simulink model "gm_sampleModel1489_sub"  (R2023a)
settings: Solver=VariableStepAuto  StartTime=0.0  StopTime=10.0  RelTol=1e-3
libraries: hdlsllib x3, simulink x1
settings Model: Creator=user1  LastModifiedBy=user1
settings OptimizationCC: BlockReduction=off  ConditionallyExecuteInputs=off
settings DebuggingCC: InheritedTsInSrcMsg=none

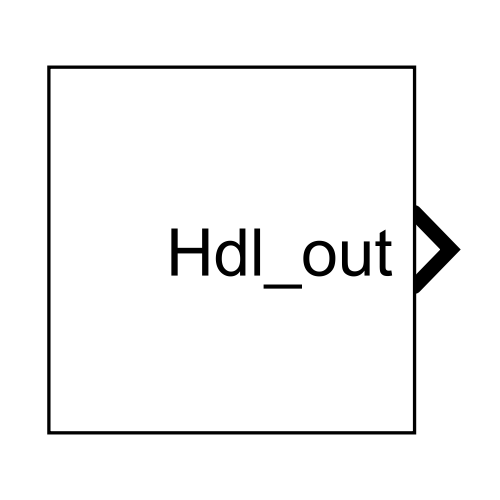
[thumbnail: Simulink's stored preview of the top-level diagram]
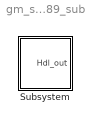
== system gm_sampleModel1489_sub ==
  Subsystem : Subsystem

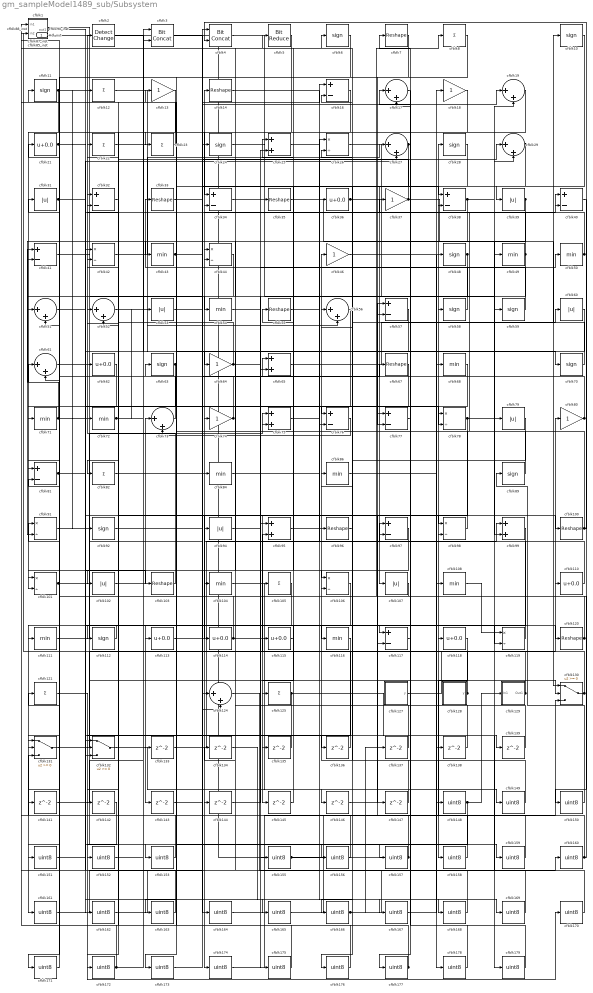
== system gm_sampleModel1489_sub/Subsystem ==
  cfblk1 : Constant  Value=0  OutDataTypeStr=uint8  SampleTime=1
  cfblk{6,10..11,24,28,48,58..59,63,70,89,92,112} (13 alike) : Signum
  cfblk{7,14,33,35,55,67,96,100,103,120} (10 alike) : Reshape
  cfblk{26,42,44,78,91,98,101,106,119} (9 alike) : Product  Inputs=*/  OutDataTypeStr=uint8  RndMeth=Zero  SaturateOnIntegerOverflow=on
  cfblk{31,39,53,60,79,94,102,107} (8 alike) : Abs  OutDataTypeStr=uint8  SaturateOnIntegerOverflow=off
  cfblk{43,49..50,54,68,71..72,84,86,104,108,111,116} (13 alike) : MinMax  OutDataTypeStr=uint8
  cfblk{8,12,22..23,82,105,121,125} (8 alike) : Sum  Inputs=+  OutDataTypeStr=uint8
  cfblk{21,36,62,110,113..115,118} (8 alike) : Bias  Bias=0.0  SaturateOnIntegerOverflow=off
  cfblk{16,32,34,38,40..41,57,76..77,81,97,117} (12 alike) : Sum  Inputs=+-  OutDataTypeStr=uint8
  cfblk{17,19,27,29,51..52,56,61,73,124} (10 alike) : Sum  Inputs=|++  OutDataTypeStr=uint8
  cfblk127 : Subsystem  mask(Counter Limited){uplimit=double(7), tsamp=double(-1)}
      mask prompts: uplimit "Simulink:masks:UpperLimit_MP"; tsamp "Simulink:masks:SampleTime_MP"
      mask help: Simulink:masks:CounterLimited_MD
      mask init:
      | nbits = double(8);
      | tsamp = double(-1);
      | uplimit = double(7);
  cfblk128 : Subsystem  mask(Counter Free-Running){NumBits=double(16), tsamp=double(-1)}
      mask prompts: NumBits "Simulink:masks:NumberOfBits_MP"; tsamp "Simulink:masks:SampleTime_MP"
      mask help: Simulink:masks:CounterFreeRunning_MD
  cfblk129 : Subsystem
  cfblk{13,18,37,46,64,74,80} (7 alike) : Gain  OutDataTypeStr=uint8
  cfblk130 : Switch  OutDataTypeStr=uint8  SaturateOnIntegerOverflow=off  InputSameDT=off
  cfblk131 : Switch  OutDataTypeStr=uint8  SaturateOnIntegerOverflow=off  InputSameDT=off
  cfblk132 : Switch  OutDataTypeStr=uint8  SaturateOnIntegerOverflow=off  InputSameDT=off
  cfblk{133..139,141..147} (14 alike) : Delay  SampleTime=1
  cfblk{148..153,155..179} (31 alike) : DataTypeConversion  OutDataTypeStr=uint8  SaturateOnIntegerOverflow=off  RndMeth=Floor
  cfblk2 : simulink/Logic and Bit Operations/Detect Change  vinit=0  OutDataTypeStr=uint8
      settings: LibrarySourceBlock=|
      | hdlsllib/Logic and Bit
      | Operations/Detect
      | Change
  cfblk{25,65,75,95,99} (5 alike) : Sum  OutDataTypeStr=uint8
  cfblk3 : hdlsllib/Logic and Bit Operations/Bit Concat  numInputs=2
  cfblk4 : hdlsllib/Logic and Bit Operations/Bit Concat  numInputs=2
  cfblk5 : hdlsllib/Logic and Bit Operations/Bit Reduce  mode=AND
  cfblk85_inst : Subsystem
  cfblk87_inst : Subsystem
  cfblk88_inst : Subsystem
  cfblk90_inst : Subsystem
  Hdl_out : Outport  OutDataTypeStr=uint8  SampleTime=1
  wires:
  cfblk1/1 -> cfblk153/1
  cfblk10/1 -> cfblk107/1
  cfblk100/1 -> cfblk4/2, cfblk28/1
  cfblk101/1 -> cfblk75/1, cfblk130/2
  cfblk102/1 -> cfblk73/1
  cfblk103/1 -> cfblk2/1
  cfblk104/1 -> cfblk146/1
  cfblk105/1 -> cfblk143/1
  cfblk106/1 -> cfblk161/1
  cfblk107/1 -> cfblk8/1
  cfblk108/1 -> cfblk119/1
  cfblk11/1 -> cfblk92/1, cfblk174/1, cfblk147/1, cfblk145/1, cfblk101/2
  cfblk110/1 -> cfblk97/1
  cfblk111/1 -> cfblk4/1
  cfblk112/1 -> cfblk111/1
  cfblk113/1 -> cfblk14/1
  cfblk114/1 -> cfblk61/2, cfblk32/1, cfblk139/1
  cfblk115/1 -> cfblk55/1
  cfblk116/1 -> cfblk135/1
  cfblk117/1 -> cfblk157/1
  cfblk118/1 -> cfblk158/1
  cfblk119/1 -> cfblk94/1
  cfblk12/1 -> cfblk56/2
  cfblk120/1 -> cfblk61/1, cfblk46/1
  cfblk121/1 -> cfblk170/1
  cfblk124/1 -> cfblk160/1
  cfblk125/1 -> cfblk179/1, cfblk144/1
  cfblk127/1(y) -> cfblk59/1
  cfblk128/1(y) -> cfblk95/2, cfblk91/1
  cfblk129/1(Out1) -> cfblk95/1, cfblk58/1, cfblk16/2
  cfblk13/1 -> cfblk112/1
  cfblk130/1 -> cfblk63/1, cfblk32/2
  cfblk131/1 -> cfblk80/1
  cfblk132/1 -> cfblk164/1
  cfblk133/1 -> cfblk26/1
  cfblk134/1 -> cfblk168/1
  cfblk135/1 -> cfblk132/2
  cfblk136/1 -> cfblk87_inst/2(in2)
  cfblk137/1 -> cfblk88_inst/2(in2)
  cfblk138/1 -> cfblk44/1
  cfblk139/1 -> cfblk98/2
  cfblk14/1 -> cfblk78/2
  cfblk141/1 -> cfblk3/2
  cfblk142/1 -> cfblk152/1
  cfblk143/1 -> cfblk29/1
  cfblk144/1 -> cfblk99/1
  cfblk145/1 -> cfblk65/1
  cfblk146/1 -> cfblk77/1
  cfblk147/1 -> cfblk106/2
  cfblk148/1 -> cfblk173/1, cfblk129/1(In1)
  cfblk149/1 -> cfblk86/1
  cfblk150/1 -> cfblk89/1
  cfblk151/1 -> cfblk40/1
  cfblk152/1 -> cfblk40/2
  cfblk153/1 -> cfblk87_inst/1(in1)
  cfblk155/1 -> cfblk130/3, cfblk18/1
  cfblk156/1 -> cfblk52/1
  cfblk157/1 -> cfblk52/2, Hdl_out/1
  cfblk158/1 -> cfblk74/1
  cfblk159/1 -> cfblk118/1
  cfblk16/1 -> cfblk34/1
  cfblk160/1 -> cfblk81/2, cfblk131/3, cfblk110/1, cfblk44/2
  cfblk161/1 -> cfblk124/1
  cfblk162/1 -> cfblk124/2
  cfblk163/1 -> cfblk21/1
  cfblk164/1 -> cfblk57/1
  cfblk165/1 -> cfblk57/2
  cfblk166/1 -> cfblk48/1, cfblk137/1, cfblk49/1
  cfblk167/1 -> cfblk68/1
  cfblk168/1 -> cfblk85_inst/1(in1)
  cfblk169/1 -> cfblk134/1
  cfblk17/1 -> cfblk177/1
  cfblk170/1 -> cfblk132/1
  cfblk171/1 -> cfblk121/1
  cfblk172/1 -> cfblk90_inst/2(in2), cfblk75/2
  cfblk173/1 -> cfblk19/1
  cfblk174/1 -> cfblk19/2
  cfblk175/1 -> cfblk85_inst/2(in2)
  cfblk176/1 -> cfblk22/1
  cfblk177/1 -> cfblk11/1, cfblk13/1
  cfblk178/1 -> cfblk17/1
  cfblk179/1 -> cfblk17/2
  cfblk18/1 -> cfblk51/1
  cfblk19/1 -> cfblk172/1
  cfblk2/1 -> cfblk64/1
  cfblk21/1 -> cfblk136/1, cfblk72/1
  cfblk22/1 -> cfblk175/1
  cfblk23/1 -> cfblk88_inst/1(in1)
  cfblk24/1 -> cfblk108/1
  cfblk25/1 -> cfblk76/2
  cfblk26/1 -> cfblk79/1
  cfblk27/1 -> cfblk117/1, cfblk105/1
  cfblk28/1 -> cfblk156/1
  cfblk29/1 -> cfblk39/1, cfblk133/1
  cfblk3/1 -> cfblk149/1
  cfblk31/1 -> cfblk162/1, cfblk98/1
  cfblk32/1 -> cfblk82/1
  cfblk33/1 -> cfblk38/1
  cfblk34/1 -> cfblk35/1
  cfblk35/1 -> cfblk99/2
  cfblk36/1 -> cfblk178/1, cfblk106/1
  cfblk37/1 -> cfblk6/1, cfblk130/1, cfblk12/1
  cfblk38/1 -> cfblk29/2, cfblk54/1
  cfblk39/1 -> cfblk41/2, cfblk91/2
  cfblk4/1 -> cfblk96/1
  cfblk40/1 -> cfblk150/1
  cfblk41/1 -> cfblk84/1
  cfblk42/1 -> cfblk27/1
  cfblk43/1 -> cfblk16/1, cfblk100/1
  cfblk44/1 -> cfblk71/1
  cfblk46/1 -> cfblk119/2
  cfblk48/1 -> cfblk65/2, cfblk131/2
  cfblk49/1 -> cfblk132/3, cfblk37/1
  cfblk5/1 -> cfblk23/1
  cfblk50/1 -> cfblk5/1, cfblk34/2
  cfblk51/1 -> cfblk114/1
  cfblk52/1 -> cfblk155/1
  cfblk53/1 -> cfblk116/1
  cfblk54/1 -> cfblk120/1
  cfblk55/1 -> cfblk36/1
  cfblk56/1 -> cfblk131/1
  cfblk57/1 -> cfblk163/1
  cfblk58/1 -> cfblk26/2
  cfblk59/1 -> cfblk33/1
  cfblk6/1 -> cfblk81/1
  cfblk60/1 -> cfblk104/1
  cfblk61/1 -> cfblk138/1
  cfblk62/1 -> cfblk151/1
  cfblk63/1 -> cfblk142/1, cfblk141/1
  cfblk64/1 -> cfblk42/2, cfblk50/1
  cfblk65/1 -> cfblk10/1
  cfblk67/1 -> cfblk113/1
  cfblk68/1 -> cfblk166/1
  cfblk7/1 -> cfblk43/1
  cfblk70/1 -> cfblk3/1
  cfblk71/1 -> cfblk41/1, cfblk165/1
  cfblk72/1 -> cfblk76/1, cfblk53/1
  cfblk73/1 -> cfblk90_inst/1(in1)
  cfblk74/1 -> cfblk51/2, cfblk31/1
  cfblk75/1 -> cfblk117/2
  cfblk76/1 -> cfblk73/2
  cfblk77/1 -> cfblk7/1
  cfblk78/1 -> cfblk60/1, cfblk102/1
  cfblk79/1 -> cfblk176/1
  cfblk8/1 -> cfblk77/2
  cfblk80/1 -> cfblk25/1, cfblk42/1
  cfblk81/1 -> cfblk27/2, cfblk101/1
  cfblk82/1 -> cfblk24/1
  cfblk84/1 -> cfblk167/1
  cfblk85_inst/1(out1) -> cfblk159/1
  cfblk86/1 -> cfblk148/1
  cfblk87_inst/1(out1) -> cfblk103/1, cfblk78/1
  cfblk88_inst/1(out1) -> cfblk70/1
  cfblk89/1 -> cfblk38/2
  cfblk90_inst/1(out1) -> cfblk169/1
  cfblk91/1 -> cfblk115/1
  cfblk92/1 -> cfblk67/1
  cfblk94/1 -> cfblk25/2
  cfblk95/1 -> cfblk97/2
  cfblk96/1 -> cfblk56/1
  cfblk97/1 -> cfblk171/1
  cfblk98/1 -> cfblk62/1
  cfblk99/1 -> cfblk125/1

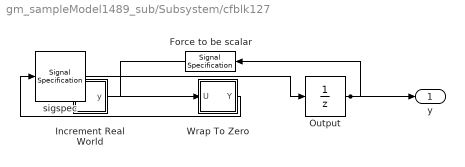
== system gm_sampleModel1489_sub/Subsystem/cfblk127 ==
  Force to be scalar : SignalSpecification  DisableCoverage=on  Dimensions=1
  Increment Real World : Subsystem  mask(Real World Value Increment){}
      mask help: Simulink:masks:RealWorldValueIncrement_MD
      mask Display: disp('V++')
  Output : UnitDelay  InitialCondition=0.0  SampleTime=tsamp  HasFrameUpgradeWarning=on
  Wrap To Zero : Subsystem  mask(Wrap To Zero){Threshold=double(7)}
      mask prompts: Threshold "Simulink:masks:Threshold_MP"
      mask help: Simulink:masks:WrapToZero_MD
  sigspec : SignalSpecification  OutDataTypeStr=uint8  Dimensions=1
  y : Outport  SampleTime=1
  wires:
  Force to be scalar/1 -> Increment Real World/1(u)
  Increment Real World/1(y) -> Wrap To Zero/1(U)
  Output/1 -> Force to be scalar/1, y/1
  Wrap To Zero/1(Y) -> sigspec/1
  sigspec/1 -> Output/1

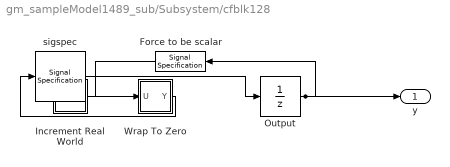
== system gm_sampleModel1489_sub/Subsystem/cfblk128 ==
  Force to be scalar : SignalSpecification  DisableCoverage=on  Dimensions=1
  Increment Real World : Subsystem  mask(Real World Value Increment){}
      mask help: Simulink:masks:RealWorldValueIncrement_MD
      mask Display: disp('V++')
  Output : UnitDelay  InitialCondition=0.0  SampleTime=tsamp  HasFrameUpgradeWarning=on
  Wrap To Zero : Subsystem  mask(Wrap To Zero){Threshold=double(65535)}
      mask prompts: Threshold "Simulink:masks:Threshold_MP"
      mask help: Simulink:masks:WrapToZero_MD
  sigspec : SignalSpecification  OutDataTypeStr=uint16  Dimensions=1
  y : Outport  SampleTime=1
  wires:
  Force to be scalar/1 -> Increment Real World/1(u)
  Increment Real World/1(y) -> Wrap To Zero/1(U)
  Output/1 -> Force to be scalar/1, y/1
  Wrap To Zero/1(Y) -> sigspec/1
  sigspec/1 -> Output/1

== system gm_sampleModel1489_sub/Subsystem/cfblk129 ==
  In1 : Inport  OutDataTypeStr=uint8  PortDimensions=1  SampleTime=1
  Out1 : Outport  SampleTime=1
  wires:
  In1/1 -> Out1/1

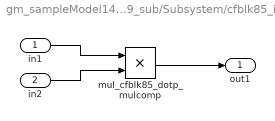
== system gm_sampleModel1489_sub/Subsystem/cfblk85_inst ==
  in1 : Inport  OutDataTypeStr=uint8  SampleTime=1
  in2 : Inport  Port=2  OutDataTypeStr=uint8  SampleTime=1
  mul_cfblk85_dotp_mulcomp : Product  Inputs=**  OutDataTypeStr=uint8  SampleTime=1
  out1 : Outport  OutDataTypeStr=uint8  SampleTime=1
  wires:
  in1/1 -> mul_cfblk85_dotp_mulcomp/1
  in2/1 -> mul_cfblk85_dotp_mulcomp/2
  mul_cfblk85_dotp_mulcomp/1 -> out1/1

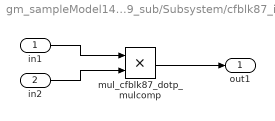
== system gm_sampleModel1489_sub/Subsystem/cfblk87_inst ==
  in1 : Inport  OutDataTypeStr=uint8  SampleTime=1
  in2 : Inport  Port=2  OutDataTypeStr=uint8  SampleTime=1
  mul_cfblk87_dotp_mulcomp : Product  Inputs=**  OutDataTypeStr=uint8  SampleTime=1
  out1 : Outport  OutDataTypeStr=uint8  SampleTime=1
  wires:
  in1/1 -> mul_cfblk87_dotp_mulcomp/1
  in2/1 -> mul_cfblk87_dotp_mulcomp/2
  mul_cfblk87_dotp_mulcomp/1 -> out1/1

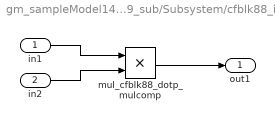
== system gm_sampleModel1489_sub/Subsystem/cfblk88_inst ==
  in1 : Inport  OutDataTypeStr=uint8  SampleTime=1
  in2 : Inport  Port=2  OutDataTypeStr=uint8  SampleTime=1
  mul_cfblk88_dotp_mulcomp : Product  Inputs=**  OutDataTypeStr=uint8  SampleTime=1
  out1 : Outport  OutDataTypeStr=uint8  SampleTime=1
  wires:
  in1/1 -> mul_cfblk88_dotp_mulcomp/1
  in2/1 -> mul_cfblk88_dotp_mulcomp/2
  mul_cfblk88_dotp_mulcomp/1 -> out1/1

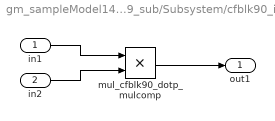
== system gm_sampleModel1489_sub/Subsystem/cfblk90_inst ==
  in1 : Inport  OutDataTypeStr=uint8  SampleTime=1
  in2 : Inport  Port=2  OutDataTypeStr=uint8  SampleTime=1
  mul_cfblk90_dotp_mulcomp : Product  Inputs=**  OutDataTypeStr=uint8  SampleTime=1
  out1 : Outport  OutDataTypeStr=uint8  SampleTime=1
  wires:
  in1/1 -> mul_cfblk90_dotp_mulcomp/1
  in2/1 -> mul_cfblk90_dotp_mulcomp/2
  mul_cfblk90_dotp_mulcomp/1 -> out1/1

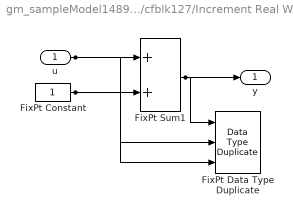
== system gm_sampleModel1489_sub/Subsystem/cfblk127/Increment Real World ==
  u : Inport  OutDataTypeStr=uint8  SampleTime=1
  FixPt Constant : Constant  DisableCoverage=on  OutDataTypeStr=Inherit: Inherit via back propagation  SampleTime=-1
  FixPt Data Type Duplicate : DataTypeDuplicate  DisableCoverage=on  NumInputPorts=3
  FixPt Sum1 : Sum  InputSameDT=on  OutDataTypeStr=Inherit: Inherit via back propagation  LockScale=on
  y : Outport  SampleTime=1
  wires:
  u/1 -> FixPt Sum1/1, FixPt Data Type Duplicate/2
  FixPt Constant/1 -> FixPt Sum1/2, FixPt Data Type Duplicate/3
  FixPt Sum1/1 -> FixPt Data Type Duplicate/1, y/1

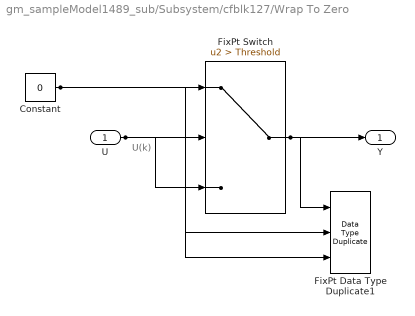
== system gm_sampleModel1489_sub/Subsystem/cfblk127/Wrap To Zero ==
  note: U(k)
  U : Inport  OutDataTypeStr=uint8  SampleTime=1
  Constant : Constant  DisableCoverage=on  Value=0  OutDataTypeStr=Inherit: Inherit via back propagation  SampleTime=-1
  FixPt Data Type Duplicate1 : DataTypeDuplicate  DisableCoverage=on  NumInputPorts=3
  FixPt Switch : Switch  Criteria=u2 > Threshold  Threshold=Threshold  OutDataTypeStr=Inherit: Inherit via back propagation  ZeroCross=off  SaturateOnIntegerOverflow=off  InputSameDT=off
  Y : Outport  SampleTime=1
  wires:
  U/1 -> FixPt Switch/3, FixPt Switch/2, FixPt Data Type Duplicate1/2
  Constant/1 -> FixPt Switch/1, FixPt Data Type Duplicate1/3
  FixPt Switch/1 -> FixPt Data Type Duplicate1/1, Y/1

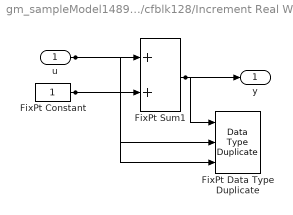
== system gm_sampleModel1489_sub/Subsystem/cfblk128/Increment Real World ==
  u : Inport  OutDataTypeStr=uint16  SampleTime=1
  FixPt Constant : Constant  DisableCoverage=on  OutDataTypeStr=Inherit: Inherit via back propagation  SampleTime=-1
  FixPt Data Type Duplicate : DataTypeDuplicate  DisableCoverage=on  NumInputPorts=3
  FixPt Sum1 : Sum  InputSameDT=on  OutDataTypeStr=Inherit: Inherit via back propagation  LockScale=on
  y : Outport  SampleTime=1
  wires:
  u/1 -> FixPt Sum1/1, FixPt Data Type Duplicate/2
  FixPt Constant/1 -> FixPt Sum1/2, FixPt Data Type Duplicate/3
  FixPt Sum1/1 -> FixPt Data Type Duplicate/1, y/1

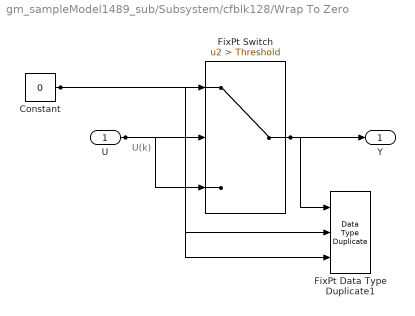
== system gm_sampleModel1489_sub/Subsystem/cfblk128/Wrap To Zero ==
  note: U(k)
  U : Inport  OutDataTypeStr=uint16  SampleTime=1
  Constant : Constant  DisableCoverage=on  Value=0  OutDataTypeStr=Inherit: Inherit via back propagation  SampleTime=-1
  FixPt Data Type Duplicate1 : DataTypeDuplicate  DisableCoverage=on  NumInputPorts=3
  FixPt Switch : Switch  Criteria=u2 > Threshold  Threshold=Threshold  OutDataTypeStr=Inherit: Inherit via back propagation  ZeroCross=off  SaturateOnIntegerOverflow=off  InputSameDT=off
  Y : Outport  SampleTime=1
  wires:
  U/1 -> FixPt Switch/3, FixPt Switch/2, FixPt Data Type Duplicate1/2
  Constant/1 -> FixPt Switch/1, FixPt Data Type Duplicate1/3
  FixPt Switch/1 -> FixPt Data Type Duplicate1/1, Y/1
